simulink model "P2PHVDCMMC"  (R2024a)
settings: Solver=FixedStepDiscrete  StartTime=0.0  StopTime=10  RelTol=1e-3
PreLoadFcn:
  | % HVDCMMCInterconnectionParam
StartFcn:
  | tic
StopFcn:
  | toc
values from neighbouring files (symbols this model uses):
  C_PM = 1.758e-3    (= 0.001758)    [P2PHVDCMMCcode.m]
  Cg = 50e-9    (= 5e-08)    [P2PHVDCMMCcode.m]
  Fc = Fnom*3.37    (= 168.5)    [P2PHVDCMMCcode.m]
  Fnom = 50    [P2PHVDCMMCcode.m]
  HRM = 1    [P2PHVDCMMCcode.m]
  Ki_Ireg = 6    [P2PHVDCMMCcode.m]
  Ki_Preg = 1.0    (= 1)    [P2PHVDCMMCcode.m]
  Ki_Qreg = 1.0    (= 1)    [P2PHVDCMMCcode.m]
  Ki_VDCreg = 100    [P2PHVDCMMCcode.m]
  Kp_Ireg = 0.6    [P2PHVDCMMCcode.m]
  Kp_Preg = 0.5/3    (= 0.166666666667)    [P2PHVDCMMCcode.m]
  Kp_Qreg = 0.5/3    (= 0.166666666667)    [P2PHVDCMMCcode.m]
  Kp_VDCreg = 4    [P2PHVDCMMCcode.m]
  L_cable = 15e-3    (= 0.015)    [P2PHVDCMMCcode.m]
  Larm = Larm_pu*(Zb_ac/(2*pi*Fnom))    [P2PHVDCMMCcode.m]
  Larm_pu = 0.15    [P2PHVDCMMCcode.m]
  Lff = Larm_pu/2    (= 0.075)    [P2PHVDCMMCcode.m]
  Limits_Ireg = [ 2.0  -2.0]    [P2PHVDCMMCcode.m]
  Limits_Preg = [ 1.2, 0.8 ]    [P2PHVDCMMCcode.m]
  Limits_Qreg = [ 0.25, -0.25 ]    [P2PHVDCMMCcode.m]
  Limits_VDCreg = [ 2.0  -2.0]    [P2PHVDCMMCcode.m]
  Lxfo = 0.12    [P2PHVDCMMCcode.m]
  N = 6    [P2PHVDCMMCcode.m]
  Nb_PM = 36    [P2PHVDCMMCcode.m]
  Pnom = 1000e6    (= 1000000000)    [P2PHVDCMMCcode.m]
  R_cable = 0.5    [P2PHVDCMMCcode.m]
  R_startup = 400    [P2PHVDCMMCcode.m]
  Rarm = Rarm_pu*Zb_ac    [P2PHVDCMMCcode.m]
  Rff = Rarm_pu/2    (= 0.00075)    [P2PHVDCMMCcode.m]
  Rg = 100    [P2PHVDCMMCcode.m]
  Rxfo = 0.003    [P2PHVDCMMCcode.m]
  Slope_Qref = 0.5    [P2PHVDCMMCcode.m]
  Slope_Vdc_ref = Vnom_dc/5    (= 128000)    [P2PHVDCMMCcode.m]
  Tfault = 9999    [P2PHVDCMMCcode.m]
  Ts = Ts_Control    (= 4e-05)    [P2PHVDCMMCcode.m]
  Ts_Control = 40e-6    (= 4e-05)    [P2PHVDCMMCcode.m]
  Ts_dqn = 2e-5    (= 2e-05)    [P2PHVDCMMCcode.m]
  Ts_Power = 20e-6    (= 2e-05)    [P2PHVDCMMCcode.m]
  Vnom_dc = 640e3    (= 640000)    [P2PHVDCMMCcode.m]
  Vnom_prim = 400e3    (= 400000)    [P2PHVDCMMCcode.m]
  Vnom_sec = 333e3    (= 333000)    [P2PHVDCMMCcode.m]
  Ws = 2*pi*50    (= 314.159265359)    [P2PHVDCMMCcode.m]
undefined symbols (not defined in the file or in its folder): DiscIntNeverNeededParam, Discrete, DQN_Lib, gcbh, Int_DQNc_Mat, Mult_DQNc_Mat, Pcc, S, sps, sps_rtmsupport, spsMeanValueVariableFrequencyModel, spsPLL3phModel, SY3
libraries: simulink x38, spsControlledVoltageSourceLib x30, spsVoltageMeasurementLib x21, spsIdealSwitchLib x21, powerlib_extras x12, spsSecondOrderFilterLib x12, spsCurrentMeasurementLib x12, spsdq0toabcLib x9, spsMeanLib x8, spsMeanVariableFrequencyLib x8, spsabctodq0Lib x8, spsThreePhaseSeriesRLCBranchLib x7
(part 1 of 13)
settings Model: SimulationMode=accelerator  Creator=The MathWorks, Inc.  LastModifiedBy=salsarayreh
settings SolverCC: AlgebraicLoopSolver=TrustRegion  AutoInsertRateTranBlk=on
settings DataIOCC: SaveFormat=StructureWithTime  SaveOutput=off  DSMLogging=off  SaveTime=off  ReturnWorkspaceOutputs=off
settings OptimizationCC: ReuseModelBlockBuffer=off  ExpressionDepthLimit=2147483647  LifeSpan=inf
settings DebuggingCC: UnderspecifiedInitializationDetection=Classic  MergeDetectMultiDrivingBlocksExec=none  SolverPrmCheckMsg=warning  MultiTaskRateTransMsg=warning  FcnCallInpInsideContextMsg=warning  UnconnectedInputMsg=warning  UnconnectedOutputMsg=warning  UnconnectedLineMsg=warning  AllowSymbolicDim=off  StateNameClashWarn=warning  SFUnexpectedBacktrackingDiag=warning  SFNoUnconditionalDefaultTransitionDiag=warning  SFExecutionAtInitializationDiag=none  ArithmeticOperatorsInVariantConditions=warning
settings HardwareCC: ProdBitPerPointer=32  ProdBitPerSizeT=32  ProdBitPerPtrDiffT=32  ProdLargestAtomicFloat=None  ProdIntDivRoundTo=Undefined  ProdEndianess=Unspecified  ProdWordSize=32  ProdHWDeviceType=32-bit Generic
settings ModelReferenceCC: EnableRefExpFcnMdlSchedulingChecks=on  PropagateSignalLabelsOutOfModel=off
settings SFSimCC: SimUseLocalCustomCode=off  CustomCodeUndefinedFunction=UseInterfaceOnly
settings RTWCC: RTWUseLocalCustomCode=off  GPUComputeCapability=3.5
settings CodeAppCC: StateflowObjectComments=on
settings GRTTargetCC: TargetLangStandard=C89/C90 (ANSI)  CombineOutputUpdateFcns=off  GRTInterface=on
settings ConfigComp: CovMetricSettings=dw  CovSaveCumulativeToWorkspaceVar=on  CovSaveSingleToWorkspaceVar=on  CovExternalEMLEnable=off
settings SimscapeCC: SimscapeNormalizeSystem=off

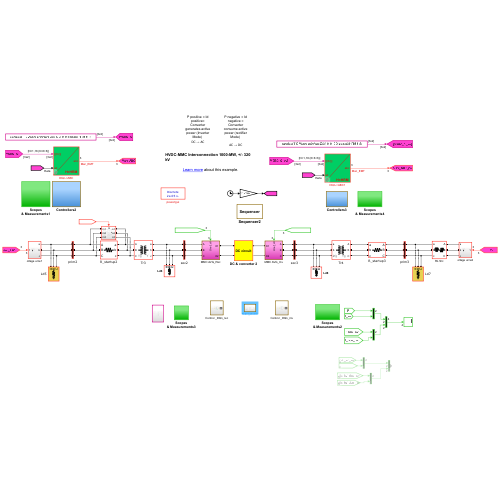
[thumbnail: Simulink's stored preview of the top-level diagram]
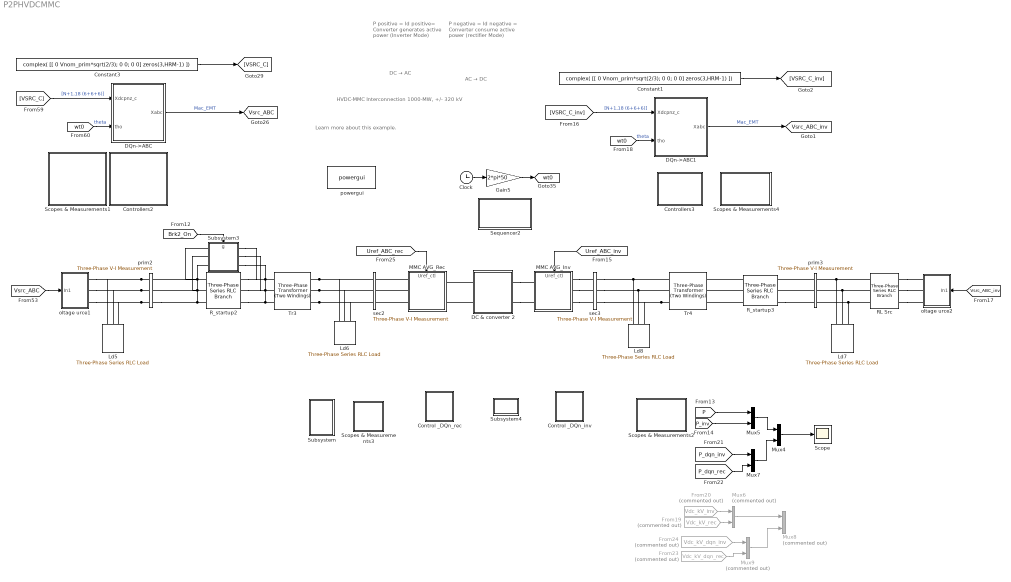
== system P2PHVDCMMC ==
  note: DC → AC
  note: HVDC-MMC Interconnection 1000-MW, +/- 320 kV
  note: Learn more about this example.
  note: P positive = Id positive= Converter generates active power (Inverter Mode)
  note: P negative = Id negative = Converter consume active power (rectifier Mode)
  note: AC → DC
  Clock : Clock
  Constant1 : Constant  Value=complex( [[ 0 Vnom_prim*sqrt(2/3); 0 0; 0 0] zeros(3,HRM-1) ])
  Constant3 : Constant  Value=complex( [[ 0 Vnom_prim*sqrt(2/3); 0 0; 0 0] zeros(3,HRM-1) ])
  Control _DQn_inv : Subsystem
  Control _DQn_rec : Subsystem
  Controllers2 : Subsystem
  Controllers3 : Subsystem
  DC & converter 2 : Subsystem
      mask Display: disp('DC circuit')
  DQn->ABC : MATLAB Function  TreatAsAtomicUnit=on  SystemSampleTime=Ts_Power  mask{N=HRM}
      mask prompts: N "Harmonic order:"
  DQn->ABC1 : MATLAB Function  TreatAsAtomicUnit=on  SystemSampleTime=Ts_Power  mask{N=HRM}
      mask prompts: N "Harmonic order:"
  From19 : From  Commented=on  GotoTag=Vdc_kV_rec  TagVisibility=global
  From20 : From  Commented=on  GotoTag=Vdc_kV_inv  TagVisibility=global
  From23 : From  Commented=on  GotoTag=Vdc_kV_dqn_rec  TagVisibility=global
  From24 : From  Commented=on  GotoTag=Vdc_kV_dqn_inv  TagVisibility=global
  Gain5 : Gain  Gain=2*pi*50
  Ld5 : spsThreePhaseSeriesRLCLoadLib/Three-Phase Series RLC Load  LConnTagsString=A|B|C  Configuration=Y (grounded)  NominalVoltage=Vnom_prim  Vabc=[1e3 1e3 1e3]  Vabcp=[1e3 1e3 1e3]  NominalFrequency=Fnom  UnbalancedPower=off  ActivePower=P_Ld1  InductivePower=0  CapacitivePower=0  Pabc=[10e3 9e3 11e3]  QLabc=[100 90 110]  QCabc=[100 90 110]  Pabcp=[10e3 9e3 11e3]  QLabcp=[100 90 110]  QCabcp=[100 90 110]  Measurements=None  LoadType=constant Z
  Ld6 : spsThreePhaseSeriesRLCLoadLib/Three-Phase Series RLC Load  LConnTagsString=A|B|C  Configuration=Y (grounded)  NominalVoltage=Vnom_sec  Vabc=[1e3 1e3 1e3]  Vabcp=[1e3 1e3 1e3]  NominalFrequency=Fnom  UnbalancedPower=off  ActivePower=500e3  InductivePower=0  CapacitivePower=0  Pabc=[10e3 9e3 11e3]  QLabc=[100 90 110]  QCabc=[100 90 110]  Pabcp=[10e3 9e3 11e3]  QLabcp=[100 90 110]  QCabcp=[100 90 110]  Measurements=None  LoadType=constant Z
  Ld7 : spsThreePhaseSeriesRLCLoadLib/Three-Phase Series RLC Load  LConnTagsString=A|B|C  Configuration=Y (grounded)  NominalVoltage=Vnom_prim  Vabc=[1e3 1e3 1e3]  Vabcp=[1e3 1e3 1e3]  NominalFrequency=Fnom  UnbalancedPower=off  ActivePower=P_Ld1  InductivePower=0  CapacitivePower=0  Pabc=[10e3 9e3 11e3]  QLabc=[100 90 110]  QCabc=[100 90 110]  Pabcp=[10e3 9e3 11e3]  QLabcp=[100 90 110]  QCabcp=[100 90 110]  Measurements=None  LoadType=constant Z
  Ld8 : spsThreePhaseSeriesRLCLoadLib/Three-Phase Series RLC Load  LConnTagsString=A|B|C  Configuration=Y (grounded)  NominalVoltage=Vnom_sec  Vabc=[1e3 1e3 1e3]  Vabcp=[1e3 1e3 1e3]  NominalFrequency=Fnom  UnbalancedPower=off  ActivePower=500e3  InductivePower=0  CapacitivePower=0  Pabc=[10e3 9e3 11e3]  QLabc=[100 90 110]  QCabc=[100 90 110]  Pabcp=[10e3 9e3 11e3]  QLabcp=[100 90 110]  QCabcp=[100 90 110]  Measurements=None  LoadType=constant Z
  MMC AVG_Inv : Subsystem
      settings: PortSchema="{\"entries\":[{\"content\":{\"sides\":[{\"content\":{\"connectorIds\":[\"LConn1\",\"LConn2\",\"LConn3\"]},\"type\":\"ConnectorPlacement.EquallySpacedRectSide\",\"uuid\":\"ba64873c-b22b-410d-af4d-7ba2fdc55c23\"},{\"content\":{\"connectorIds\":[\"RConn1\",\"RConn2\"],\"side\":\"RIGHT\"},\"type\":\"ConnectorPlacement.EquallySpacedRectSide\",\"uuid\":\"193af711-64d0-4e3f-b9d8-3af97f0f6abc\"},{\"content\":{\"connectorIds\":[\"In1\"],\"side\":\"TOP\"},\"type\":\"ConnectorPlacement.EquallySpacedRectSide\",\"uuid\":\"04826a8d-a462-403d-873f-6ac7e8481113\"}]},\"type\":\"ConnectorPlacement.EquallySpacedConnector\",\"uuid\":\"1def47fd-2da9-40af-b501-c2103dcb1fab\"}],\"packageUris\":[\"http://schema.mathworks.com/mf0/Connector/R2020b\"],\"version\":\"1.0\"}"
  MMC AVG_Rec : Subsystem
      settings: PortSchema="{\"entries\":[{\"content\":{\"sides\":[{\"content\":{\"connectorIds\":[\"LConn1\",\"LConn2\",\"LConn3\"]},\"type\":\"ConnectorPlacement.EquallySpacedRectSide\",\"uuid\":\"ba64873c-b22b-410d-af4d-7ba2fdc55c23\"},{\"content\":{\"connectorIds\":[\"RConn1\",\"RConn2\"],\"side\":\"RIGHT\"},\"type\":\"ConnectorPlacement.EquallySpacedRectSide\",\"uuid\":\"193af711-64d0-4e3f-b9d8-3af97f0f6abc\"},{\"content\":{\"connectorIds\":[\"In1\"],\"side\":\"TOP\"},\"type\":\"ConnectorPlacement.EquallySpacedRectSide\",\"uuid\":\"04826a8d-a462-403d-873f-6ac7e8481113\"}]},\"type\":\"ConnectorPlacement.EquallySpacedConnector\",\"uuid\":\"1def47fd-2da9-40af-b501-c2103dcb1fab\"}],\"packageUris\":[\"http://schema.mathworks.com/mf0/Connector/R2020b\"],\"version\":\"1.0\"}"
  Mux4 : Mux  Inputs=2
  Mux5 : Mux  Inputs=2
  Mux6 : Mux  Commented=on  Inputs=2
  Mux7 : Mux  Inputs=2
  Mux8 : Mux  Commented=on  Inputs=2
  Mux9 : Mux  Commented=on  Inputs=2
  RL Src : spsThreePhaseSeriesRLCBranchLib/Three-Phase Series RLC Branch  LConnTagsString=A|B|C  RConnTagsString=A|B|C  BranchType=RL  Resistance=0.8929  Inductance=16.58e-3  Capacitance=1e-6  Measurements=None
  R_startup2 : spsThreePhaseSeriesRLCBranchLib/Three-Phase Series RLC Branch  LConnTagsString=A|B|C  RConnTagsString=A|B|C  BranchType=R  Resistance=R_startup  Inductance=Vnom_prim^2 / Pcc / (2*pi*Fnom)  Capacitance=1e-6  Measurements=None
  R_startup3 : spsThreePhaseSeriesRLCBranchLib/Three-Phase Series RLC Branch  LConnTagsString=A|B|C  RConnTagsString=A|B|C  BranchType=R  Resistance=R_startup/5  Inductance=Vnom_prim^2 / Pcc / (2*pi*Fnom)  Capacitance=1e-6  Measurements=None
  Scope : Scope
  Scopes & Measurements1 : Subsystem
  Scopes & Measurements2 : Subsystem
  Scopes & Measurements3 : Subsystem
  Scopes & Measurements4 : Subsystem
  Sequencer2 : Subsystem
      mask Display: disp('Sequencer')
  Subsystem : Subsystem
  Subsystem3 : Subsystem
      settings: PortSchema="{\"entries\":[{\"content\":{\"sides\":[{\"content\":{\"connectorIds\":[\"LConn1\",\"LConn2\",\"LConn3\"]},\"type\":\"ConnectorPlacement.EquallySpacedRectSide\",\"uuid\":\"c1a766f8-ff9e-46aa-a021-7821e1e68416\"},{\"content\":{\"connectorIds\":[\"RConn1\",\"RConn2\",\"RConn3\"],\"side\":\"RIGHT\"},\"type\":\"ConnectorPlacement.EquallySpacedRectSide\",\"uuid\":\"987c4934-70c2-4017-a470-918577d5d1f5\"},{\"content\":{\"connectorIds\":[\"In1\"],\"side\":\"TOP\"},\"type\":\"ConnectorPlacement.EquallySpacedRectSide\",\"uuid\":\"288129dd-9593-42f2-8eec-9a4ff51cc6bc\"}]},\"type\":\"ConnectorPlacement.EquallySpacedConnector\",\"uuid\":\"6c6a961f-0497-41f0-a1bb-4cb9411a874b\"}],\"packageUris\":[\"http://schema.mathworks.com/mf0/Connector/R2020b\"],\"version\":\"1.0\"}"
  Subsystem4 : Subsystem
  Tr3 : spsThreePhaseTransformerTwoWindingsLib/Three-Phase Transformer (Two Windings)  Winding1Connection=Yg  Winding2Connection=Y  CoreType=Three single-phase transformers  SetSaturation=off  Hysteresis=off  DataFile='hysteresis'  SetInitialFlux=off  Measurements=None  UNITS=pu  NominalPower=[ Pnom , Fnom ]  Winding1="[ Vnom_prim , Rxfo/2,  Lxfo/2 ]"  Winding2="[ Vnom_sec , Rxfo/2,  Lxfo/2 ]"  Rm=1000  Lm=1000  L0=0.5  Saturation=[ 0,0 ; 0.0024,1.2 ; 1.0,1.52 ]  InitialFluxes=[ 0.8 , -0.8 , 0.7 ]  BreakLoop=off  DiscreteSolver=Trapezoidal iterative  DataType=off  TransfoNumber=1
  Tr4 : spsThreePhaseTransformerTwoWindingsLib/Three-Phase Transformer (Two Windings)  Winding1Connection=Yg  Winding2Connection=Yg  CoreType=Three single-phase transformers  SetSaturation=off  Hysteresis=off  DataFile='hysteresis'  SetInitialFlux=off  Measurements=None  UNITS=pu  NominalPower=[ Pnom , Fnom ]  Winding1="[ Vnom_prim , Rxfo/2,  Lxfo/2 ]"  Winding2="[ Vnom_sec , Rxfo/2,  Lxfo/2 ]"  Rm=1000  Lm=1000  L0=0.5  Saturation=[ 0,0 ; 0.0024,1.2 ; 1.0,1.52 ]  InitialFluxes=[ 0.8 , -0.8 , 0.7 ]  BreakLoop=off  DiscreteSolver=Trapezoidal iterative  DataType=off  TransfoNumber=1
  oltage urce1 : Subsystem
  oltage urce2 : Subsystem
  powergui : spspowerguiLib/powergui  Priority=1  SimulationMode=Discrete  SampleTime=Ts_Power  frequency=60  Iterations=50  frequencyindice=0  Pbase=100e6  ErrMax=1e-4  UnitsV=kV  UnitsW=MW  buscounter=0  FunctionMessages=off  echomessages=off  EnableUseOfTLC=off  CurrentSourceSwitches=off  DisableSnubberDevices=off  DisableRonSwitches=off  DisableVfSwitches=off  DisplayEquations=off  AutomaticDiscreteSolvers=off  SolverType=Tustin/Backward Euler (TBE)  Interpol=off  ExternalGateDelay=off  methode=off  Ts=10  x0status=blocks  SPID=off  SwTol=0  HookPort=off  NonlinearTolerance=1e-4  nMaxIteration=100  ContinueOnMaxIteration=off  RestoreLinks=warning  ResistiveCurrentMeasurement=off  Frange=[0:2:500]  Ylog=off  Xlog=on  ShowGrid=off  save=off  variable=ZData  structure=VIprim  ZoomFFT=on  StartTime=0.15  cycles=2  DisplayStyle=1  fundamental=50  FreqAxis=on  MaxFrequency=1000  frequencyindicesteady=1  RmsSteady=1  display=off
  prim2 : spsThreePhaseVIMeasurementLib/Three-Phase V-I Measurement  VoltageMeasurement=phase-to-ground  SetLabelV=on  LabelV=Vprim  Vpu=off  VpuLL=off  CurrentMeasurement=yes  SetLabelI=on  LabelI=Iprim  Ipu=off  Pbase=100e6  Vbase=500e3  OutputType=Complex  PhasorSimulation=off  PSBequivalent=0
  prim3 : spsThreePhaseVIMeasurementLib/Three-Phase V-I Measurement  VoltageMeasurement=phase-to-ground  SetLabelV=on  LabelV=Vprim_inv  Vpu=off  VpuLL=off  CurrentMeasurement=yes  SetLabelI=on  LabelI=Iprim_inv  Ipu=off  Pbase=100e6  Vbase=500e3  OutputType=Complex  PhasorSimulation=off  PSBequivalent=0
  sec2 : spsThreePhaseVIMeasurementLib/Three-Phase V-I Measurement  VoltageMeasurement=phase-to-ground  SetLabelV=on  LabelV=Vsec  Vpu=off  VpuLL=off  CurrentMeasurement=yes  SetLabelI=on  LabelI=Isec  Ipu=off  Pbase=100e6  Vbase=500e3  OutputType=Complex  PhasorSimulation=off  PSBequivalent=0
  sec3 : spsThreePhaseVIMeasurementLib/Three-Phase V-I Measurement  VoltageMeasurement=phase-to-ground  SetLabelV=on  LabelV=Vsec_inv  Vpu=off  VpuLL=off  CurrentMeasurement=yes  SetLabelI=on  LabelI=Isec_inv  Ipu=off  Pbase=100e6  Vbase=500e3  OutputType=Complex  PhasorSimulation=off  PSBequivalent=0
  tag scope: Vsrc_ABC=global, Vsrc_ABC_inv=global, wt0=global
  wires:
  [Vsrc_ABC] -> oltage urce1/1(In1)
  Gain5/1 -> [wt0]
  [Uref_ABC_rec] -> MMC AVG_Rec/1(Uref_ctl)
  [VSRC_C] -> DQn->ABC/1(Xdcpnz_c)  "[N+1,18 (6+6+6)]"
  [wt0] -> DQn->ABC/2(tho)  "theta"
  Constant3/1 -> [VSRC_C]
  Clock/1 -> Gain5/1
  DQn->ABC/1(Xabc) -> [Vsrc_ABC]  "Mac_EMT"
  [Brk2_On] -> Subsystem3/1(g)
  [Vsrc_ABC_inv] -> oltage urce2/1(In1)
  [Uref_ABC_inv] -> MMC AVG_Inv/1(Uref_ctl)
  [wt0] -> DQn->ABC1/2(tho)  "theta"
  Constant1/1 -> [VSRC_C_inv]
  [VSRC_C_inv] -> DQn->ABC1/1(Xdcpnz_c)  "[N+1,18 (6+6+6)]"
  DQn->ABC1/1(Xabc) -> [Vsrc_ABC_inv]  "Mac_EMT"
  [P] -> Mux5/1
  [P_inv] -> Mux5/2
  Mux5/1 -> Mux4/1
  Mux4/1 -> Scope/1
  Mux6/1 -> Mux8/1
  From19/1 -> Mux6/2
  From20/1 -> Mux6/1
  [P_dqn_rec] -> Mux7/2
  [P_dqn_inv] -> Mux7/1
  Mux7/1 -> Mux4/2
  From24/1 -> Mux9/1
  From23/1 -> Mux9/2
  Mux9/1 -> Mux8/2
  connections:
  Tr3/RConn2 -- sec2/RConn2 -- Ld6/LConn2
  Tr3/RConn1 -- sec2/RConn1 -- Ld6/LConn1
  Tr3/RConn3 -- sec2/RConn3 -- Ld6/LConn3
  Tr3/LConn2 -- Subsystem3/RConn2 -- R_startup2/RConn2
  R_startup2/LConn2 -- Subsystem3/LConn2 -- prim2/LConn2
  R_startup2/LConn3 -- Subsystem3/LConn3 -- prim2/LConn3
  Tr3/LConn1 -- Subsystem3/RConn1 -- R_startup2/RConn1
  Tr3/LConn3 -- Subsystem3/RConn3 -- R_startup2/RConn3
  R_startup2/LConn1 -- Subsystem3/LConn1 -- prim2/LConn1
  prim2/RConn1 -- Ld5/LConn1 -- oltage urce1/RConn1
  prim2/RConn3 -- Ld5/LConn3 -- oltage urce1/RConn3
  prim2/RConn2 -- Ld5/LConn2 -- oltage urce1/RConn2
  MMC AVG_Rec/LConn1 -- sec2/LConn1
  DC & converter 2/LConn2 -- MMC AVG_Rec/RConn2
  MMC AVG_Rec/LConn2 -- sec2/LConn2
  MMC AVG_Rec/LConn3 -- sec2/LConn3
  DC & converter 2/LConn1 -- MMC AVG_Rec/RConn1
  Tr4/RConn3 -- sec3/RConn3 -- Ld8/LConn3
  RL Src/RConn1 -- Ld7/LConn1 -- prim3/RConn1
  prim3/LConn2 -- R_startup3/LConn2
  RL Src/RConn3 -- Ld7/LConn3 -- prim3/RConn3
  R_startup3/RConn1 -- Tr4/LConn1
  R_startup3/RConn3 -- Tr4/LConn3
  RL Src/RConn2 -- Ld7/LConn2 -- prim3/RConn2
  sec3/RConn1 -- Ld8/LConn1 -- Tr4/RConn1
  R_startup3/LConn3 -- prim3/LConn3
  prim3/LConn1 -- R_startup3/LConn1
  R_startup3/RConn2 -- Tr4/LConn2
  sec3/RConn2 -- Ld8/LConn2 -- Tr4/RConn2
  RL Src/LConn3 -- oltage urce2/RConn3
  MMC AVG_Inv/LConn2 -- sec3/LConn2
  MMC AVG_Inv/LConn3 -- sec3/LConn3
  MMC AVG_Inv/LConn1 -- sec3/LConn1
  RL Src/LConn1 -- oltage urce2/RConn1
  RL Src/LConn2 -- oltage urce2/RConn2
  DC & converter 2/RConn1 -- MMC AVG_Inv/RConn1
  DC & converter 2/RConn2 -- MMC AVG_Inv/RConn2

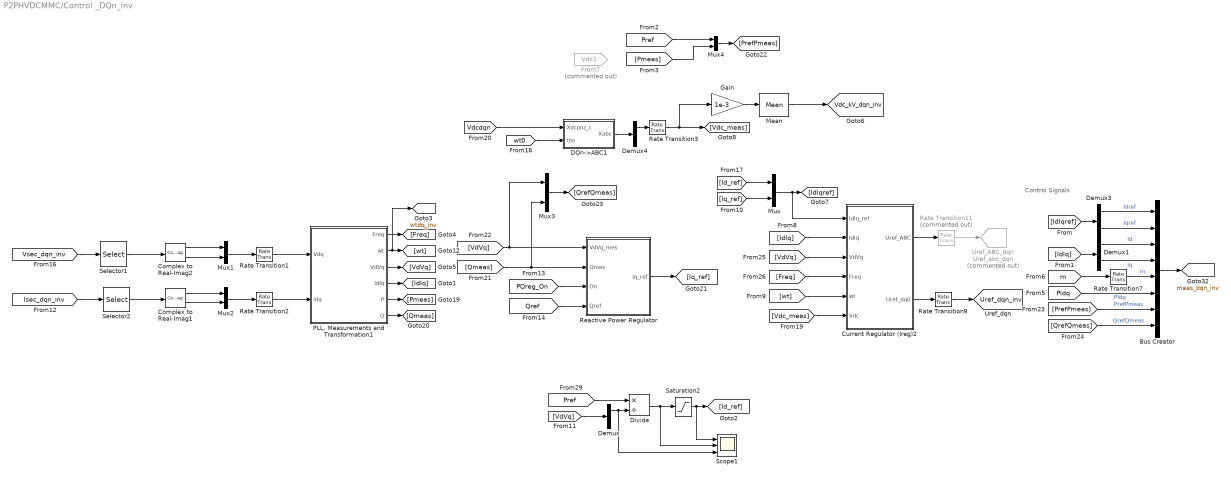
== system P2PHVDCMMC/Control _DQn_inv ==
  note: Control Signals
  Bus Creator : BusCreator  Inputs=8
  Complex to Real-Imag1 : ComplexToRealImag
  Complex to Real-Imag2 : ComplexToRealImag
  Current Regulator (Ireg)2 : Subsystem
  DQn->ABC1 : MATLAB Function  TreatAsAtomicUnit=on  SystemSampleTime=Ts_Power  mask{N=N+3}
      mask prompts: N "Harmonic order:"
  Demux : Demux  Outputs=2
  Demux1 : Demux  Outputs=2
  Demux3 : Demux  Outputs=2
  Demux4 : Demux  Outputs=3
  Divide : Product  Inputs=*/
  From7 : From  Commented=on  GotoTag=Vdc1  TagVisibility=global
  Gain : Gain  Gain=1e-3
  Mean : spsMeanLib/Mean  Freq=Fnom/3  Vinit=0  Ts=Ts_Control
  Mux{,1..4} (5 alike) : Mux  Inputs=2
  "PLL, Measurements and Transformation1" : Subsystem
  Rate Transition{1..3,7} (4 alike) : RateTransition  OutPortSampleTime=Ts_Control
  Rate Transition11 : RateTransition  Commented=on  OutPortSampleTime=Ts_Power
  Rate Transition9 : RateTransition  OutPortSampleTime=Ts_Power
  Reactive Power Regulator : Subsystem
  Saturation2 : Saturate  UpperLimit=Limits_VDCreg(1)  LowerLimit=Limits_VDCreg(2)  SampleTime=Ts
  Scope1 : Scope  NumInputPorts=3
  Selector1 : Selector  NumberOfDimensions=2  InputPortWidth=3  IndexOptions=Index vector (dialog),Index vector (dialog)  Indices=1,2  OutputSizes=1,1
  Selector2 : Selector  NumberOfDimensions=2  InputPortWidth=3  IndexOptions=Index vector (dialog),Index vector (dialog)  Indices=1,2  OutputSizes=1,1
  Uref_ABC_dqn : Goto  Commented=on  GotoTag=Uref_abc_dqn  TagVisibility=global
  tag scope: Uref_dqn_inv=global, Vdc_kV_dqn_inv=global, meas_dqn_inv=global, wtdq_inv=global
  wires:
  Complex to Real-Imag2/1 -> Mux1/1
  [PQreg_On] -> Reactive Power Regulator/3(On)
  Selector1/1 -> Complex to Real-Imag2/1
  Complex to Real-Imag2/2 -> Mux1/2
  [Vsec_dqn_inv] -> Selector1/1
  [Qref] -> Reactive Power Regulator/4(Qref)
  Complex to Real-Imag1/2 -> Mux2/2
  Selector2/1 -> Complex to Real-Imag1/1
  Complex to Real-Imag1/1 -> Mux2/1
  [Isec_dqn_inv] -> Selector2/1
  Current Regulator (Ireg)2/1(Uref_ABC) -> Rate Transition11/1
  Mux1/1 -> Rate Transition1/1
  Mux2/1 -> Rate Transition2/1
  Rate Transition1/1 -> "PLL, Measurements and Transformation1"/1(Vdq)
  Rate Transition2/1 -> "PLL, Measurements and Transformation1"/2(Idq)
  Rate Transition11/1 -> Uref_ABC_dqn/1
  [PrefPmeas] -> Bus Creator/7  "PrefPmeas"
  [Pref] -> Mux4/1
  [QrefQmeas] -> Bus Creator/8  "QrefQmeas"
  Mux4/1 -> [PrefPmeas]
  Gain/1 -> Mean/1
  [Pmeas] -> Mux4/2
  [m] -> Rate Transition7/1
  Rate Transition3/1 -> Gain/1, [Vdc_meas]
  Demux3/1 -> Bus Creator/1  "Idref"
  Rate Transition7/1 -> Bus Creator/5  "m"
  [IdIq] -> Demux1/1
  Bus Creator/1 -> [meas_dqn_inv]
  Demux1/1 -> Bus Creator/3  "Id"
  Demux3/2 -> Bus Creator/2  "Iqref"
  [IdIqref] -> Demux3/1
  [PIdq] -> Bus Creator/6  "PIdq"
  [Id_ref] -> Mux/1
  Demux1/2 -> Bus Creator/4  "Iq"
  [Iq_ref] -> Mux/2
  Mean/1 -> [Vdc_kV_dqn_inv]
  "PLL, Measurements and Transformation1"/6(Q) -> [Qmeas]
  "PLL, Measurements and Transformation1"/5(P) -> [Pmeas]
  "PLL, Measurements and Transformation1"/4(IdIq) -> [IdIq]
  "PLL, Measurements and Transformation1"/3(VdVq) -> [VdVq]
  "PLL, Measurements and Transformation1"/2(wt) -> [wtdq_inv], [wt]
  "PLL, Measurements and Transformation1"/1(Freq) -> [Freq]
  Reactive Power Regulator/1(Iq_ref) -> [Iq_ref]
  [Qmeas] -> Mux3/2, Reactive Power Regulator/2(Qmes)
  [VdVq] -> Mux3/1, Reactive Power Regulator/1(VdVq_mes)
  Mux3/1 -> [QrefQmeas]
  Mux/1 -> Current Regulator (Ireg)2/1(IdIq_ref), [IdIqref]
  [IdIq] -> Current Regulator (Ireg)2/2(IdIq)
  [VdVq] -> Current Regulator (Ireg)2/3(VdVq)
  [wt] -> Current Regulator (Ireg)2/5(wt)
  [Freq] -> Current Regulator (Ireg)2/4(Freq)
  [Vdc_meas] -> Current Regulator (Ireg)2/6(Vdc)
  Current Regulator (Ireg)2/2(Uref_dq0) -> Rate Transition9/1
  Rate Transition9/1 -> [Uref_dqn_inv]
  Demux/1 -> Scope1/3, Divide/2
  Saturation2/1 -> Scope1/1, [Id_ref]
  Divide/1 -> Scope1/2, Saturation2/1
  [Pref] -> Divide/1
  [VdVq] -> Demux/1
  [wt0] -> DQn->ABC1/2(tho)
  Demux4/1 -> Rate Transition3/1
  [Vdcdqn] -> DQn->ABC1/1(Xdcpnz_c)
  DQn->ABC1/1(Xabc) -> Demux4/1

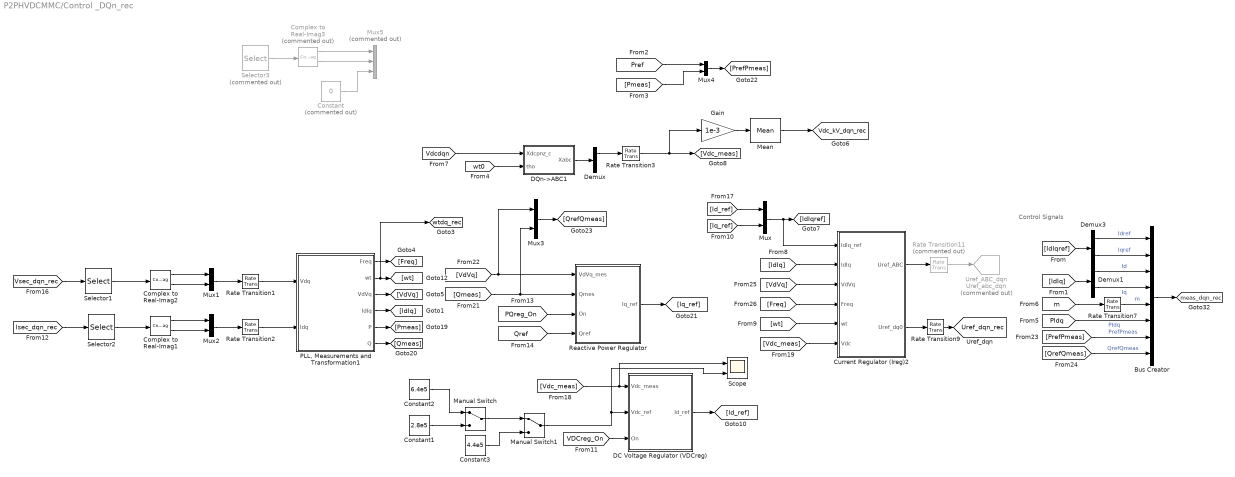
== system P2PHVDCMMC/Control _DQn_rec ==
  note: Control Signals
  Bus Creator : BusCreator  Inputs=8
  Complex to Real-Imag1 : ComplexToRealImag
  Complex to Real-Imag2 : ComplexToRealImag
  Complex to Real-Imag3 : ComplexToRealImag  Commented=on
  Constant : Constant  Commented=on  Value=0
  Constant1 : Constant  Value=2.8e5  SampleTime=Ts_Control
  Constant2 : Constant  Value=6.4e5  SampleTime=Ts_Control
  Constant3 : Constant  Value=4.4e5  SampleTime=Ts_Control
  Current Regulator (Ireg)2 : Subsystem
  DC Voltage Regulator (VDCreg) : Subsystem
  DQn->ABC1 : MATLAB Function  TreatAsAtomicUnit=on  SystemSampleTime=Ts_Power  mask{N=N+3}
      mask prompts: N "Harmonic order:"
  Demux : Demux  Outputs=3
  Demux1 : Demux  Outputs=2
  Demux3 : Demux  Outputs=2
  Gain : Gain  Gain=1e-3
  Manual Switch : ManualSwitch
  Manual Switch1 : ManualSwitch
  Mean : spsMeanLib/Mean  Freq=Fnom/3  Vinit=0  Ts=Ts_Control
  Mux{,1..4} (5 alike) : Mux  Inputs=2
  Mux5 : Mux  Commented=on  Inputs=3
  "PLL, Measurements and Transformation1" : Subsystem
  Rate Transition{1..3,7} (4 alike) : RateTransition  OutPortSampleTime=Ts_Control
  Rate Transition11 : RateTransition  Commented=on  OutPortSampleTime=Ts_Power
  Rate Transition9 : RateTransition  OutPortSampleTime=Ts_Power
  Reactive Power Regulator : Subsystem
  Scope : Scope  NumInputPorts=2
  Selector1 : Selector  NumberOfDimensions=2  InputPortWidth=3  IndexOptions=Index vector (dialog),Index vector (dialog)  Indices=1,2  OutputSizes=1,1
  Selector2 : Selector  NumberOfDimensions=2  InputPortWidth=3  IndexOptions=Index vector (dialog),Index vector (dialog)  Indices=1,2  OutputSizes=1,1
  Selector3 : Selector  Commented=on  NumberOfDimensions=2  InputPortWidth=3  IndexOptions=Index vector (dialog),Index vector (dialog)  Indices=3,1  OutputSizes=1,1
  Uref_ABC_dqn : Goto  Commented=on  GotoTag=Uref_abc_dqn  TagVisibility=global
  tag scope: Uref_dqn_rec=global, Vdc_kV_dqn_rec=global, meas_dqn_rec=global, wtdq_rec=global
  wires:
  Complex to Real-Imag2/1 -> Mux1/1
  [PQreg_On] -> Reactive Power Regulator/3(On)
  Selector1/1 -> Complex to Real-Imag2/1
  Complex to Real-Imag2/2 -> Mux1/2
  [Vsec_dqn_rec] -> Selector1/1
  [Qref] -> Reactive Power Regulator/4(Qref)
  Complex to Real-Imag1/2 -> Mux2/2
  Selector2/1 -> Complex to Real-Imag1/1
  Complex to Real-Imag1/1 -> Mux2/1
  [Isec_dqn_rec] -> Selector2/1
  Current Regulator (Ireg)2/1(Uref_ABC) -> Rate Transition11/1
  Mux1/1 -> Rate Transition1/1
  Mux2/1 -> Rate Transition2/1
  Rate Transition1/1 -> "PLL, Measurements and Transformation1"/1(Vdq)
  Rate Transition2/1 -> "PLL, Measurements and Transformation1"/2(Idq)
  Rate Transition11/1 -> Uref_ABC_dqn/1
  [PrefPmeas] -> Bus Creator/7  "PrefPmeas"
  [Pref] -> Mux4/1
  [QrefQmeas] -> Bus Creator/8  "QrefQmeas"
  Mux4/1 -> [PrefPmeas]
  Gain/1 -> Mean/1
  [Pmeas] -> Mux4/2
  [m] -> Rate Transition7/1
  Rate Transition3/1 -> Gain/1, [Vdc_meas]
  Demux3/1 -> Bus Creator/1  "Idref"
  Rate Transition7/1 -> Bus Creator/5  "m"
  [IdIq] -> Demux1/1
  Bus Creator/1 -> [meas_dqn_rec]
  Demux1/1 -> Bus Creator/3  "Id"
  Demux3/2 -> Bus Creator/2  "Iqref"
  [IdIqref] -> Demux3/1
  [PIdq] -> Bus Creator/6  "PIdq"
  [Id_ref] -> Mux/1
  Demux1/2 -> Bus Creator/4  "Iq"
  DQn->ABC1/1(Xabc) -> Demux/1
  [Iq_ref] -> Mux/2
  Mean/1 -> [Vdc_kV_dqn_rec]
  "PLL, Measurements and Transformation1"/6(Q) -> [Qmeas]
  "PLL, Measurements and Transformation1"/5(P) -> [Pmeas]
  "PLL, Measurements and Transformation1"/4(IdIq) -> [IdIq]
  "PLL, Measurements and Transformation1"/3(VdVq) -> [VdVq]
  "PLL, Measurements and Transformation1"/2(wt) -> [wtdq_rec], [wt]
  "PLL, Measurements and Transformation1"/1(Freq) -> [Freq]
  Reactive Power Regulator/1(Iq_ref) -> [Iq_ref]
  [Qmeas] -> Mux3/2, Reactive Power Regulator/2(Qmes)
  [VdVq] -> Mux3/1, Reactive Power Regulator/1(VdVq_mes)
  Mux3/1 -> [QrefQmeas]
  Mux/1 -> Current Regulator (Ireg)2/1(IdIq_ref), [IdIqref]
  [IdIq] -> Current Regulator (Ireg)2/2(IdIq)
  [VdVq] -> Current Regulator (Ireg)2/3(VdVq)
  [wt] -> Current Regulator (Ireg)2/5(wt)
  [Freq] -> Current Regulator (Ireg)2/4(Freq)
  [Vdc_meas] -> Current Regulator (Ireg)2/6(Vdc)
  Current Regulator (Ireg)2/2(Uref_dq0) -> Rate Transition9/1
  Rate Transition9/1 -> [Uref_dqn_rec]
  Constant3/1 -> Manual Switch1/2
  Constant1/1 -> Manual Switch/2
  Constant2/1 -> Manual Switch/1
  DC Voltage Regulator (VDCreg)/1(Id_ref) -> [Id_ref]
  Manual Switch/1 -> Manual Switch1/1
  [Vdc_meas] -> Scope/1, DC Voltage Regulator (VDCreg)/1(Vdc_meas)
  Manual Switch1/1 -> Scope/2, DC Voltage Regulator (VDCreg)/2(Vdc_ref)
  [VDCreg_On] -> DC Voltage Regulator (VDCreg)/3(On)
  Complex to Real-Imag3/1 -> Mux5/1
  Complex to Real-Imag3/2 -> Mux5/2
  Selector3/1 -> Complex to Real-Imag3/1
  [Vdcdqn] -> DQn->ABC1/1(Xdcpnz_c)
  Constant/1 -> Mux5/3
  Demux/1 -> Rate Transition3/1
  [wt0] -> DQn->ABC1/2(tho)

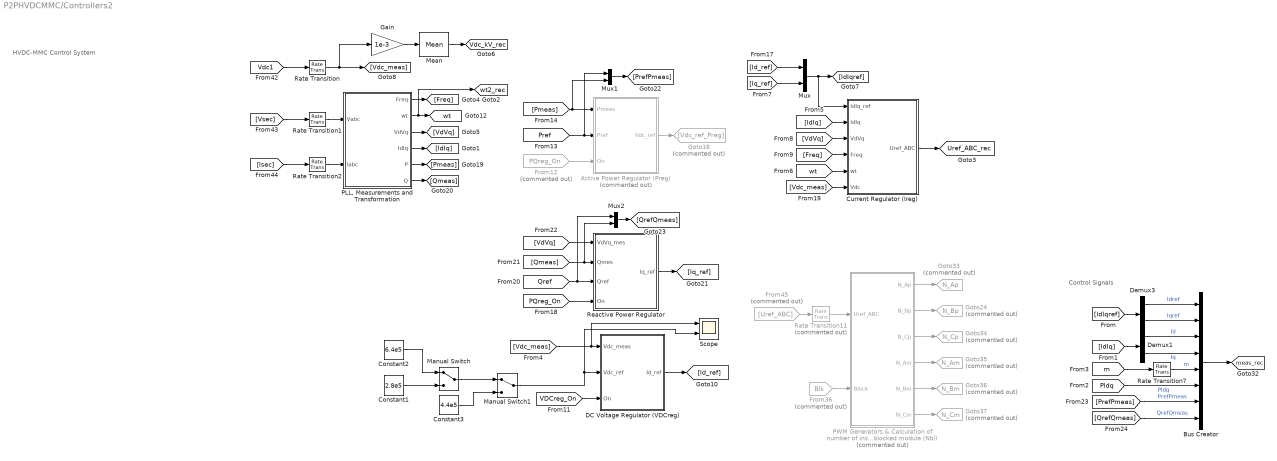
== system P2PHVDCMMC/Controllers2 ==
  note: HVDC-MMC Control System
  note: Control Signals
  Active Power Regulator (Preg) : Subsystem  Commented=on
  Bus Creator : BusCreator  Inputs=8
  Constant1 : Constant  Value=2.8e5  SampleTime=Ts_Control
  Constant2 : Constant  Value=6.4e5  SampleTime=Ts_Control
  Constant3 : Constant  Value=4.4e5  SampleTime=Ts_Control
  Current Regulator (Ireg) : Subsystem
  DC Voltage Regulator (VDCreg) : Subsystem
  Demux1 : Demux  Outputs=2
  Demux3 : Demux  Outputs=2
  From12 : From  Commented=on  GotoTag=PQreg_On  TagVisibility=global
  From36 : From  Commented=on  GotoTag=Blk  TagVisibility=global
  From45 : From  Commented=on  GotoTag=Uref_ABC  TagVisibility=global
  Gain : Gain  Gain=1e-3
  Goto18 : Goto  Commented=on  GotoTag=Vdc_ref_Preg
  Goto24 : Goto  Commented=on  GotoTag=N_Bp  TagVisibility=global
  Goto33 : Goto  Commented=on  GotoTag=N_Ap  TagVisibility=global
  Goto34 : Goto  Commented=on  GotoTag=N_Cp  TagVisibility=global
  Goto35 : Goto  Commented=on  GotoTag=N_Am  TagVisibility=global
  Goto36 : Goto  Commented=on  GotoTag=N_Bm  TagVisibility=global
  Goto37 : Goto  Commented=on  GotoTag=N_Cm  TagVisibility=global
  Manual Switch : ManualSwitch
  Manual Switch1 : ManualSwitch
  Mean : spsMeanLib/Mean  Freq=Fnom/3  Vinit=0  Ts=Ts_Control
  Mux : Mux  Inputs=2
  Mux1 : Mux  Inputs=2
  Mux2 : Mux  Inputs=2
  "PLL, Measurements and Transformation" : Subsystem
  PWM Generators & Calculation of number of inserted modules (Nin) and number of blocked module (Nbl) : Subsystem  Commented=on
  Rate Transition{,1..2,7} (4 alike) : RateTransition  OutPortSampleTime=Ts_Control
  Rate Transition11 : RateTransition  Commented=on  OutPortSampleTime=Ts_Power
  Reactive Power Regulator : Subsystem
  Scope : Scope  NumInputPorts=2
  tag scope: Uref_ABC_rec=global, Vdc_kV_rec=global, meas_rec=global, wt2_rec=global, wt=global
  wires:
  Rate Transition11/1 -> PWM Generators & Calculation of number of inserted modules (Nin) and number of blocked module (Nbl)/1(Uref_ABC)
  From45/1 -> Rate Transition11/1
  Mean/1 -> [Vdc_kV_rec]
  [Vsec] -> Rate Transition1/1
  [Isec] -> Rate Transition2/1
  [Vdc_meas] -> Current Regulator (Ireg)/6(Vdc)
  [Vdc_meas] -> Scope/1, DC Voltage Regulator (VDCreg)/1(Vdc_meas)
  DC Voltage Regulator (VDCreg)/1(Id_ref) -> [Id_ref]
  Gain/1 -> Mean/1
  Current Regulator (Ireg)/1(Uref_ABC) -> [Uref_ABC_rec]
  [wt] -> Current Regulator (Ireg)/5(wt)
  [Vdc1] -> Rate Transition/1
  "PLL, Measurements and Transformation"/2(wt) -> [wt], [wt2_rec]
  "PLL, Measurements and Transformation"/4(IdIq) -> [IdIq]
  [Freq] -> Current Regulator (Ireg)/4(Freq)
  [Id_ref] -> Mux/1
  "PLL, Measurements and Transformation"/3(VdVq) -> [VdVq]
  Mux/1 -> Current Regulator (Ireg)/1(IdIq_ref), [IdIqref]
  Demux1/2 -> Bus Creator/4  "Iq"
  [IdIq] -> Current Regulator (Ireg)/2(IdIq)
  [IdIqref] -> Demux3/1
  Demux3/1 -> Bus Creator/1  "Idref"
  [IdIq] -> Demux1/1
  Bus Creator/1 -> [meas_rec]
  Demux3/2 -> Bus Creator/2  "Iqref"
  [m] -> Rate Transition7/1
  Demux1/1 -> Bus Creator/3  "Id"
  [PIdq] -> Bus Creator/6  "PIdq"
  "PLL, Measurements and Transformation"/1(Freq) -> [Freq]
  [VdVq] -> Current Regulator (Ireg)/3(VdVq)
  [Iq_ref] -> Mux/2
  Rate Transition/1 -> Gain/1, [Vdc_meas]
  Rate Transition2/1 -> "PLL, Measurements and Transformation"/2(Iabc)
  Rate Transition7/1 -> Bus Creator/5  "m"
  Rate Transition1/1 -> "PLL, Measurements and Transformation"/1(Vabc)
  [PQreg_On] -> Reactive Power Regulator/4(On)
  Mux2/1 -> [QrefQmeas]
  Mux1/1 -> [PrefPmeas]
  [Qref] -> Mux2/1, Reactive Power Regulator/3(Qref)
  [QrefQmeas] -> Bus Creator/8  "QrefQmeas"
  [VDCreg_On] -> DC Voltage Regulator (VDCreg)/3(On)
  From12/1 -> Active Power Regulator (Preg)/3(On)
  Active Power Regulator (Preg)/1(Vdc_ref) -> Goto18/1
  Reactive Power Regulator/1(Iq_ref) -> [Iq_ref]
  "PLL, Measurements and Transformation"/5(P) -> [Pmeas]
  [VdVq] -> Reactive Power Regulator/1(VdVq_mes)
  [Qmeas] -> Mux2/2, Reactive Power Regulator/2(Qmes)
  [Pref] -> Active Power Regulator (Preg)/2(Pref), Mux1/1
  [PrefPmeas] -> Bus Creator/7  "PrefPmeas"
  "PLL, Measurements and Transformation"/6(Q) -> [Qmeas]
  [Pmeas] -> Active Power Regulator (Preg)/1(Pmeas), Mux1/2
  PWM Generators & Calculation of number of inserted modules (Nin) and number of blocked module (Nbl)/1(N_Ap) -> Goto33/1
  PWM Generators & Calculation of number of inserted modules (Nin) and number of blocked module (Nbl)/2(N_Bp) -> Goto24/1
  PWM Generators & Calculation of number of inserted modules (Nin) and number of blocked module (Nbl)/3(N_Cp) -> Goto34/1
  PWM Generators & Calculation of number of inserted modules (Nin) and number of blocked module (Nbl)/4(N_Am) -> Goto35/1
  PWM Generators & Calculation of number of inserted modules (Nin) and number of blocked module (Nbl)/5(N_Bm) -> Goto36/1
  PWM Generators & Calculation of number of inserted modules (Nin) and number of blocked module (Nbl)/6(N_Cm) -> Goto37/1
  From36/1 -> PWM Generators & Calculation of number of inserted modules (Nin) and number of blocked module (Nbl)/2(Block)
  Manual Switch1/1 -> Scope/2, DC Voltage Regulator (VDCreg)/2(Vdc_ref)
  Constant2/1 -> Manual Switch/1
  Constant1/1 -> Manual Switch/2
  Manual Switch/1 -> Manual Switch1/1
  Constant3/1 -> Manual Switch1/2

== system P2PHVDCMMC/Controllers3 ==
  note: Control Signals
  Bus Creator : BusCreator  Inputs=8
  Constant : Constant  Commented=on  Value=6.4e5
  Current Regulator (Ireg) : Subsystem
  Demux : Demux  Outputs=2
  Demux1 : Demux  Outputs=2
  Demux3 : Demux  Outputs=2
  Divide : Product  Inputs=*/
  Gain : Gain  Gain=1e-3
  Goto9 : Goto  Commented=on  GotoTag=Uref_ABC_dq2  TagVisibility=global
  Mean : spsMeanLib/Mean  Freq=Fnom/3  Vinit=0  Ts=Ts_Control
  Mux : Mux  Inputs=2
  Mux1 : Mux  Inputs=2
  Mux2 : Mux  Inputs=2
  "PLL, Measurements and Transformation" : Subsystem
  Rate Transition{,1..2,7} (4 alike) : RateTransition  OutPortSampleTime=Ts_Control
  Reactive Power Regulator : Subsystem
  Saturation2 : Saturate  UpperLimit=Limits_VDCreg(1)  LowerLimit=Limits_VDCreg(2)  SampleTime=Ts
  Scope1 : Scope  Commented=on
  tag scope: Uref_ABC_inv=global, Vdc_kV_inv=global, meas_inv=global, wt2_inv=global
  wires:
  Mean/1 -> [Vdc_kV_inv]
  [Vsec_inv] -> Rate Transition1/1
  [Isec_inv] -> Rate Transition2/1
  [Vdc_meas] -> Current Regulator (Ireg)/6(Vdc)
  Gain/1 -> Mean/1
  Current Regulator (Ireg)/1(Uref_ABC) -> [Uref_ABC_inv]
  [wt] -> Current Regulator (Ireg)/5(wt)
  [Vdc1] -> Rate Transition/1
  "PLL, Measurements and Transformation"/2(wt) -> [wt2_inv], [wt]
  "PLL, Measurements and Transformation"/4(IdIq) -> [IdIq]
  [Freq] -> Current Regulator (Ireg)/4(Freq)
  [Id_ref] -> Mux/1
  "PLL, Measurements and Transformation"/3(VdVq) -> [VdVq]
  Mux/1 -> Current Regulator (Ireg)/1(IdIq_ref), [IdIqref]
  Demux1/2 -> Bus Creator/4  "Iq"
  [IdIq] -> Current Regulator (Ireg)/2(IdIq)
  [IdIqref] -> Demux3/1
  Demux3/1 -> Bus Creator/1  "Idref"
  [IdIq] -> Demux1/1
  Bus Creator/1 -> [meas_inv]
  Demux3/2 -> Bus Creator/2  "Iqref"
  [m_inv] -> Rate Transition7/1
  Demux1/1 -> Bus Creator/3  "Id"
  [PIdq_inv] -> Bus Creator/6  "PIdq"
  "PLL, Measurements and Transformation"/1(Freq) -> [Freq]
  [VdVq] -> Current Regulator (Ireg)/3(VdVq)
  [Iq_ref] -> Mux/2
  Rate Transition/1 -> Gain/1, [Vdc_meas]
  Rate Transition2/1 -> "PLL, Measurements and Transformation"/2(Iabc)
  Rate Transition7/1 -> Bus Creator/5  "m"
  Rate Transition1/1 -> "PLL, Measurements and Transformation"/1(Vabc)
  [PQreg_On] -> Reactive Power Regulator/4(On)
  Mux2/1 -> [QrefQmeas]
  Mux1/1 -> [PrefPmeas]
  [Qref] -> Mux2/1, Reactive Power Regulator/3(Qref)
  [QrefQmeas] -> Bus Creator/8  "QrefQmeas"
  Reactive Power Regulator/1(Iq_ref) -> [Iq_ref]
  "PLL, Measurements and Transformation"/5(P) -> [Pmeas]
  [VdVq] -> Reactive Power Regulator/1(VdVq_mes)
  [Qmeas] -> Mux2/2, Reactive Power Regulator/2(Qmes)
  [Pref] -> Mux1/1
  [PrefPmeas] -> Bus Creator/7  "PrefPmeas"
  "PLL, Measurements and Transformation"/6(Q) -> [Qmeas]
  [Pmeas] -> Mux1/2
  [Pref] -> Divide/1
  Demux/1 -> Divide/2
  Divide/1 -> Scope1/1, Saturation2/1
  [VdVq] -> Demux/1
  Saturation2/1 -> [Id_ref]
  Current Regulator (Ireg)/2(Uref_dq0) -> Goto9/1

== system P2PHVDCMMC/DC & converter 2 ==
  note: Cable (simplified model)
  CnDC : spsSeriesRLCBranchLib/Series RLC Branch  LConnTagsString=__new0  RConnTagsString=__new0  BranchType=RC  Resistance=Rg  Inductance=1e-3  SetiL0=off  InitialCurrent=0  Capacitance=Cg  Setx0=off  InitialVoltage=Vnom_dc/2  Measurements=None
  CpDC : spsSeriesRLCBranchLib/Series RLC Branch  LConnTagsString=__new0  RConnTagsString=__new0  BranchType=RC  Resistance=Rg  Inductance=1e-3  SetiL0=off  InitialCurrent=0  Capacitance=Cg  Setx0=off  InitialVoltage=Vnom_dc/2  Measurements=None
  Ground4 : spsGroundLib/Ground  LConnTagsString=a
  Subsystem : Subsystem
      settings: PortSchema="{\"entries\":[{\"content\":{\"sides\":[{\"content\":{},\"type\":\"ConnectorPlacement.EquallySpacedRectSide\",\"uuid\":\"4e02d665-d085-4b85-80a9-e764fc967845\"},{\"content\":{\"side\":\"RIGHT\"},\"type\":\"ConnectorPlacement.EquallySpacedRectSide\",\"uuid\":\"30de6932-84d3-45b2-9250-05848cfa24a7\"},{\"content\":{\"connectorIds\":[\"LConn1\"],\"side\":\"TOP\"},\"type\":\"ConnectorPlacement.EquallySpacedRectSide\",\"uuid\":\"b576265a-02ae-4a0d-b102-a95af34a8809\"},{\"content\":{\"connectorIds\":[\"RConn1\"],\"side\":\"BOTTOM\"},\"type\":\"ConnectorPlacement.EquallySpacedRectSide\",\"uuid\":\"0a0a1a6f-d60d-4cd9-8e89-b506a5f99912\"}]},\"type\":\"ConnectorPlacement.EquallySpacedConnector\",\"uuid\":\"a940d721-c0be-496a-91aa-f93d82b250c4\"}],\"packageUris\":[\"http://schema.mathworks.com/mf0/Connector/R2020b\"],\"version\":\"1.0\"}"
  Zcable1_1 : spsSeriesRLCBranchLib/Series RLC Branch  LConnTagsString=__new0  RConnTagsString=__new0  BranchType=RL  Resistance=R_cable/2  Inductance=L_cable/2  SetiL0=off  InitialCurrent=0  Capacitance=1e-6  Setx0=off  InitialVoltage=0  Measurements=None
  Zcable1_2 : spsSeriesRLCBranchLib/Series RLC Branch  LConnTagsString=__new0  RConnTagsString=__new0  BranchType=RL  Resistance=R_cable/2  Inductance=L_cable/2  SetiL0=off  InitialCurrent=0  Capacitance=1e-6  Setx0=off  InitialVoltage=0  Measurements=None
  Zcable2_1 : spsSeriesRLCBranchLib/Series RLC Branch  LConnTagsString=__new0  RConnTagsString=__new0  BranchType=RL  Resistance=R_cable/2  Inductance=L_cable/2  SetiL0=off  InitialCurrent=0  Capacitance=1e-6  Setx0=off  InitialVoltage=0  Measurements=None
  Zcable2_2 : spsSeriesRLCBranchLib/Series RLC Branch  LConnTagsString=__new0  RConnTagsString=__new0  BranchType=RL  Resistance=R_cable/2  Inductance=L_cable/2  SetiL0=off  InitialCurrent=0  Capacitance=1e-6  Setx0=off  InitialVoltage=0  Measurements=None
  1 : PMIOPort  Side=Left
  2 : PMIOPort  Port=2  Side=Left
  Connection Port : PMIOPort  Port=3  Side=Right
  Connection Port1 : PMIOPort  Port=4  Side=Right
  connections:
  Ground4/LConn1 -- CnDC/LConn1 -- CpDC/RConn1
  Subsystem/LConn1 -- Zcable1_1/RConn1 -- CpDC/LConn1 -- 1/RConn1
  CnDC/RConn1 -- 2/RConn1 -- Zcable2_1/RConn1 -- Subsystem/RConn1
  Zcable1_1/LConn1 -- Zcable1_2/RConn1
  Zcable2_2/RConn1 -- Zcable2_1/LConn1
  Connection Port/RConn1 -- Zcable1_2/LConn1
  Connection Port1/RConn1 -- Zcable2_2/LConn1

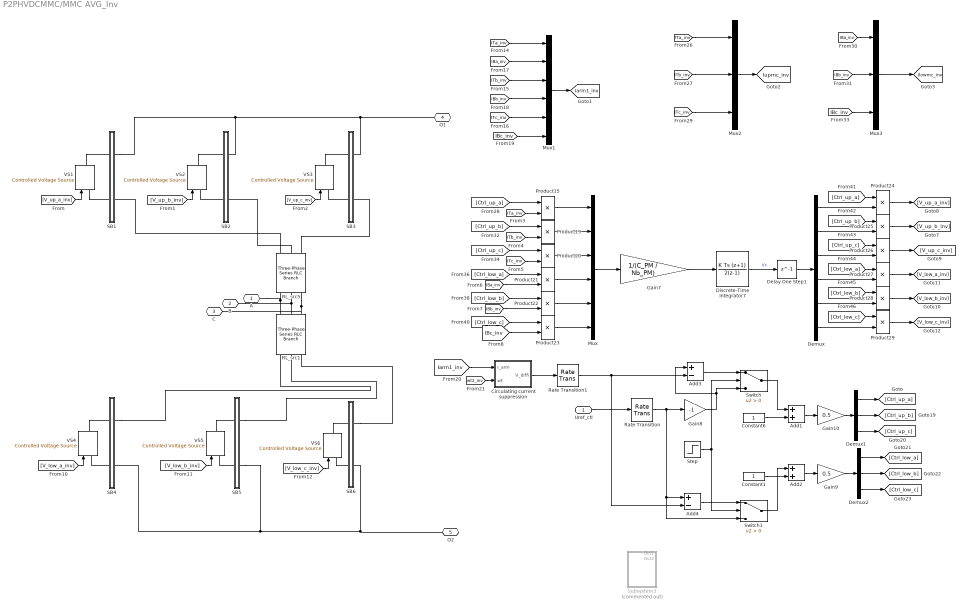
== system P2PHVDCMMC/MMC AVG_Inv ==
  Uref_ctl : Inport
  Add1 : Sum
  Add2 : Sum
  Add3 : Sum  Inputs=+-
  Add4 : Sum  Inputs=+-
  Circulating current suppression : Subsystem  VariantControl=Variant1
  Constant1 : Constant
  Constant6 : Constant
  Delay One Step1 : Delay  DelayLength=1
  Demux : Demux  Outputs=6
  Demux1 : Demux  Outputs=3
  Demux2 : Demux  Outputs=3
  Discrete-Time Integrator7 : DiscreteIntegrator  IntegratorMethod=Integration: Trapezoidal  gainval=1  SampleTime=Ts_Power  UpperSaturationLimit=5000  LowerSaturationLimit=500  ICPrevOutput=DiscIntNeverNeededParam  ICPrevScaledInput=DiscIntNeverNeededParam
  Gain10 : Gain  Gain=0.5
  Gain7 : Gain  Gain=1/(C_PM / Nb_PM)
  Gain8 : Gain  Gain=-1
  Gain9 : Gain  Gain=0.5
  Mux : Mux  Inputs=6
  Mux1 : Mux  Inputs=6
  Mux2 : Mux  Inputs=3
  Mux3 : Mux  Inputs=3
  Product{15,19..29} (12 alike) : Product
  RL_src1 : spsThreePhaseSeriesRLCBranchLib/Three-Phase Series RLC Branch  LConnTagsString=A|B|C  RConnTagsString=A|B|C  BranchType=RL  Resistance=Rarm  Inductance=Larm  Capacitance=1/(0.55*0.080*(500e3^2/100e6))/(2*pi*60)  Measurements=None
  RL_src5 : spsThreePhaseSeriesRLCBranchLib/Three-Phase Series RLC Branch  LConnTagsString=A|B|C  RConnTagsString=A|B|C  BranchType=RL  Resistance=Rarm  Inductance=Larm  Capacitance=1/(0.55*0.080*(500e3^2/100e6))/(2*pi*60)  Measurements=None
  Rate Transition : RateTransition  OutPortSampleTime=Ts_Power
  Rate Transition1 : RateTransition  OutPortSampleTime=Ts_Power
  SB1 : Subsystem
  SB2 : Subsystem
  SB3 : Subsystem
  SB4 : Subsystem
  SB5 : Subsystem
  SB6 : Subsystem
  Step : Step  Time=2  SampleTime=0
  Subsystem3 : Subsystem  Commented=on
  Switch : Switch  Criteria=u2 > Threshold  SaturateOnIntegerOverflow=off  InputSameDT=off
  Switch1 : Switch  Criteria=u2 > Threshold  SaturateOnIntegerOverflow=off  InputSameDT=off
  VS{1..6} (6 alike) : spsControlledVoltageSourceLib/Controlled Voltage Source  Initialize=on  Source_Type=AC  Amplitude=0  Phase=0  Frequency=0  Measurements=None
  A : PMIOPort  Side=Left
  B : PMIOPort  Port=2  Side=Left
  C : PMIOPort  Port=3  Side=Left
  O1 : PMIOPort  Port=4  Side=Right
  O2 : PMIOPort  Port=5  Side=Right
  tag scope: Iarm1_inv=global, Ilowmc_inv=global, Iupmc_inv=global
  wires:
  Add4/1 -> Switch1/1
  Gain8/1 -> Switch/3, Add3/1
  Add3/1 -> Switch/1
  Rate Transition1/1 -> Add4/2, Add3/2
  [IBa_inv] -> Mux1/2
  Circulating current suppression/1(V_diffi) -> Rate Transition1/1
  Mux1/1 -> [Iarm1_inv]
  [IBc_inv] -> Mux1/6
  [IBb_inv] -> Mux1/4
  Product29/1 -> [V_low_c_inv]
  Constant6/1 -> Add1/2
  Uref_ctl/1 -> Rate Transition/1
  Demux/5 -> Product28/2
  Demux2/2 -> [Ctrl_low_b]
  Product25/1 -> [V_up_b_inv]
  [Ctrl_low_b] -> Product22/1
  Product20/1 -> Mux/3
  Constant1/1 -> Add2/2
  [Ctrl_low_a] -> Product27/1
  Demux1/2 -> [Ctrl_up_b]
  [Ctrl_up_b] -> Product25/1
  Gain9/1 -> Demux2/1
  Demux/6 -> Product29/2
  Gain10/1 -> Demux1/1
  Demux/3 -> Product26/2
  [Ctrl_up_a] -> Product24/1
  Product28/1 -> [V_low_b_inv]
  Demux2/1 -> [Ctrl_low_a]
  [Ctrl_up_c] -> Product26/1
  Product23/1 -> Mux/6
  Demux1/3 -> [Ctrl_up_c]
  Product19/1 -> Mux/2
  [Ctrl_up_c] -> Product20/1
  [Ctrl_low_a] -> Product21/1
  [Ctrl_up_b] -> Product19/1
  [Ctrl_low_c] -> Product23/1
  [Ctrl_up_a] -> Product15/1
  Product27/1 -> [V_low_a_inv]
  Rate Transition/1 -> Gain8/1, Switch1/3, Add4/1
  Discrete-Time Integrator7/1 -> Delay One Step1/1  "Vc"
  Demux/4 -> Product27/2
  Add2/1 -> Gain9/1
  Product21/1 -> Mux/4
  Demux1/1 -> [Ctrl_up_a]
  Step/1 -> Switch/2, Switch1/2
  [ITa_inv] -> Mux1/1
  [ITc_inv] -> Mux1/5
  Product22/1 -> Mux/5
  Mux/1 -> Gain7/1
  Demux2/3 -> [Ctrl_low_c]
  Delay One Step1/1 -> Demux/1
  Product26/1 -> [V_up_c_inv]
  Demux/2 -> Product25/2
  [Ctrl_low_c] -> Product29/1
  Product15/1 -> Mux/1
  [Ctrl_low_b] -> Product28/1
  Product24/1 -> [V_up_a_inv]
  Add1/1 -> Gain10/1
  [wt2_inv] -> Circulating current suppression/2(wt)
  [ITb_inv] -> Mux1/3
  [Iarm1_inv] -> Circulating current suppression/1(I_arm)
  Demux/1 -> Product24/2
  Gain7/1 -> Discrete-Time Integrator7/1
  [V_up_c_inv] -> VS3/1
  [V_low_a_inv] -> VS4/1
  [V_up_a_inv] -> VS1/1
  [V_low_b_inv] -> VS5/1
  [V_up_b_inv] -> VS2/1
  [V_low_c_inv] -> VS6/1
  [ITa_inv] -> Product15/2
  [ITc_inv] -> Product20/2
  [ITb_inv] -> Product19/2
  [IBa_inv] -> Product21/2
  [IBb_inv] -> Product22/2
  [IBc_inv] -> Product23/2
  [ITb_inv] -> Mux2/2
  [ITc_inv] -> Mux2/3
  [ITa_inv] -> Mux2/1
  Mux2/1 -> [Iupmc_inv]
  [IBa_inv] -> Mux3/1
  [IBb_inv] -> Mux3/2
  [IBc_inv] -> Mux3/3
  Mux3/1 -> [Ilowmc_inv]
  Switch1/1 -> Add2/1
  Switch/1 -> Add1/1
  connections:
  VS1/LConn1 -- SB1/LConn2
  SB5/LConn2 -- VS5/LConn1
  RL_src5/LConn2 -- SB2/RConn2
  SB3/LConn1 -- VS3/RConn1
  SB4/LConn2 -- VS4/LConn1
  SB2/LConn1 -- VS2/RConn1
  SB5/RConn1 -- RL_src1/LConn2
  SB6/LConn1 -- VS6/RConn1
  SB6/RConn1 -- RL_src1/LConn3
  SB4/RConn1 -- RL_src1/LConn1
  VS1/RConn1 -- SB1/LConn1
  SB4/LConn1 -- VS4/RConn1
  RL_src5/LConn3 -- SB3/RConn2
  SB5/LConn1 -- VS5/RConn1
  VS6/LConn1 -- SB6/LConn2
  SB3/LConn2 -- VS3/LConn1
  SB2/LConn2 -- VS2/LConn1
  RL_src1/RConn1 -- A/RConn1 -- RL_src5/RConn1
  RL_src1/RConn2 -- RL_src5/RConn2 -- B/RConn1
  RL_src1/RConn3 -- RL_src5/RConn3 -- C/RConn1
  RL_src5/LConn1 -- SB1/RConn2
  SB3/RConn1 -- SB2/RConn1 -- SB1/RConn1 -- O1/RConn1
  O2/RConn1 -- SB6/RConn2 -- SB5/RConn2 -- SB4/RConn2

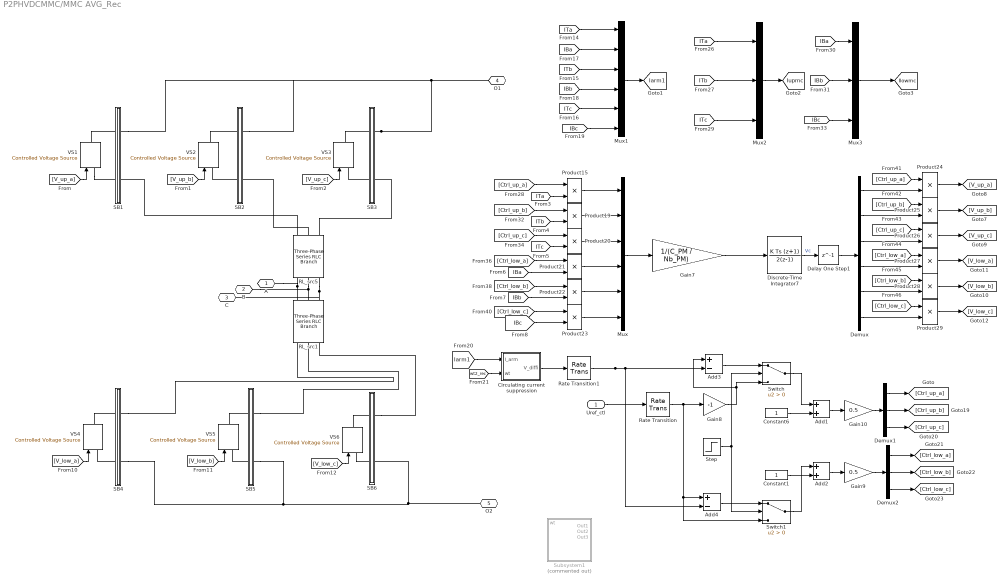
== system P2PHVDCMMC/MMC AVG_Rec ==
  Uref_ctl : Inport
  Add1 : Sum
  Add2 : Sum
  Add3 : Sum  Inputs=+-
  Add4 : Sum  Inputs=+-
  Circulating current suppression : Subsystem  VariantControl=Variant1
  Constant1 : Constant
  Constant6 : Constant
  Delay One Step1 : Delay  DelayLength=1
  Demux : Demux  Outputs=6
  Demux1 : Demux  Outputs=3
  Demux2 : Demux  Outputs=3
  Discrete-Time Integrator7 : DiscreteIntegrator  IntegratorMethod=Integration: Trapezoidal  gainval=1  SampleTime=Ts_Power  UpperSaturationLimit=5000  LowerSaturationLimit=500  ICPrevOutput=DiscIntNeverNeededParam  ICPrevScaledInput=DiscIntNeverNeededParam
  Gain10 : Gain  Gain=0.5
  Gain7 : Gain  Gain=1/(C_PM / Nb_PM)
  Gain8 : Gain  Gain=-1
  Gain9 : Gain  Gain=0.5
  Mux : Mux  Inputs=6
  Mux1 : Mux  Inputs=6
  Mux2 : Mux  Inputs=3
  Mux3 : Mux  Inputs=3
  Product{15,19..29} (12 alike) : Product
  RL_src1 : spsThreePhaseSeriesRLCBranchLib/Three-Phase Series RLC Branch  LConnTagsString=A|B|C  RConnTagsString=A|B|C  BranchType=RL  Resistance=Rarm  Inductance=Larm  Capacitance=1/(0.55*0.080*(500e3^2/100e6))/(2*pi*60)  Measurements=None
  RL_src5 : spsThreePhaseSeriesRLCBranchLib/Three-Phase Series RLC Branch  LConnTagsString=A|B|C  RConnTagsString=A|B|C  BranchType=RL  Resistance=Rarm  Inductance=Larm  Capacitance=1/(0.55*0.080*(500e3^2/100e6))/(2*pi*60)  Measurements=None
  Rate Transition : RateTransition  OutPortSampleTime=Ts_Power
  Rate Transition1 : RateTransition  OutPortSampleTime=Ts_Power
  SB1 : Subsystem
  SB2 : Subsystem
  SB3 : Subsystem
  SB4 : Subsystem
  SB5 : Subsystem
  SB6 : Subsystem
  Step : Step  Time=2  SampleTime=0
  Subsystem1 : Subsystem  Commented=on
  Switch : Switch  Criteria=u2 > Threshold  SaturateOnIntegerOverflow=off  InputSameDT=off
  Switch1 : Switch  Criteria=u2 > Threshold  SaturateOnIntegerOverflow=off  InputSameDT=off
  VS{1..6} (6 alike) : spsControlledVoltageSourceLib/Controlled Voltage Source  Initialize=on  Source_Type=AC  Amplitude=0  Phase=0  Frequency=0  Measurements=None
  A : PMIOPort  Side=Left
  B : PMIOPort  Port=2  Side=Left
  C : PMIOPort  Port=3  Side=Left
  O1 : PMIOPort  Port=4  Side=Right
  O2 : PMIOPort  Port=5  Side=Right
  tag scope: Iarm1=global, Ilowmc=global, Iupmc=global
  wires:
  Add4/1 -> Switch1/1
  Gain8/1 -> Switch/3, Add3/1
  Add3/1 -> Switch/1
  Rate Transition1/1 -> Add4/2, Add3/2
  [IBa] -> Mux1/2
  Circulating current suppression/1(V_diffi) -> Rate Transition1/1
  Mux1/1 -> [Iarm1]
  [IBc] -> Mux1/6
  [IBb] -> Mux1/4
  Product29/1 -> [V_low_c]
  Constant6/1 -> Add1/2
  Uref_ctl/1 -> Rate Transition/1
  Demux/5 -> Product28/2
  Demux2/2 -> [Ctrl_low_b]
  Product25/1 -> [V_up_b]
  [Ctrl_low_b] -> Product22/1
  Product20/1 -> Mux/3
  Constant1/1 -> Add2/2
  [Ctrl_low_a] -> Product27/1
  Demux1/2 -> [Ctrl_up_b]
  [Ctrl_up_b] -> Product25/1
  Gain9/1 -> Demux2/1
  Demux/6 -> Product29/2
  Gain10/1 -> Demux1/1
  Demux/3 -> Product26/2
  [Ctrl_up_a] -> Product24/1
  Product28/1 -> [V_low_b]
  Demux2/1 -> [Ctrl_low_a]
  [Ctrl_up_c] -> Product26/1
  Product23/1 -> Mux/6
  Demux1/3 -> [Ctrl_up_c]
  Product19/1 -> Mux/2
  [Ctrl_up_c] -> Product20/1
  [Ctrl_low_a] -> Product21/1
  [Ctrl_up_b] -> Product19/1
  [Ctrl_low_c] -> Product23/1
  [Ctrl_up_a] -> Product15/1
  Product27/1 -> [V_low_a]
  Rate Transition/1 -> Gain8/1, Switch1/3, Add4/1
  Discrete-Time Integrator7/1 -> Delay One Step1/1  "Vc"
  Demux/4 -> Product27/2
  Add2/1 -> Gain9/1
  Product21/1 -> Mux/4
  Demux1/1 -> [Ctrl_up_a]
  Step/1 -> Switch/2, Switch1/2
  [ITa] -> Mux1/1
  [ITc] -> Mux1/5
  Product22/1 -> Mux/5
  Mux/1 -> Gain7/1
  Demux2/3 -> [Ctrl_low_c]
  Delay One Step1/1 -> Demux/1
  Product26/1 -> [V_up_c]
  Demux/2 -> Product25/2
  [Ctrl_low_c] -> Product29/1
  Product15/1 -> Mux/1
  [Ctrl_low_b] -> Product28/1
  Product24/1 -> [V_up_a]
  Add1/1 -> Gain10/1
  [wt2_rec] -> Circulating current suppression/2(wt)
  [ITb] -> Mux1/3
  [Iarm1] -> Circulating current suppression/1(I_arm)
  Demux/1 -> Product24/2
  Gain7/1 -> Discrete-Time Integrator7/1
  [V_up_c] -> VS3/1
  [V_low_a] -> VS4/1
  [V_up_a] -> VS1/1
  [V_low_b] -> VS5/1
  [V_up_b] -> VS2/1
  [V_low_c] -> VS6/1
  [ITa] -> Product15/2
  [ITc] -> Product20/2
  [ITb] -> Product19/2
  [IBa] -> Product21/2
  [IBb] -> Product22/2
  [IBc] -> Product23/2
  [ITb] -> Mux2/2
  [ITc] -> Mux2/3
  [ITa] -> Mux2/1
  Mux2/1 -> [Iupmc]
  [IBa] -> Mux3/1
  [IBb] -> Mux3/2
  [IBc] -> Mux3/3
  Mux3/1 -> [Ilowmc]
  Switch1/1 -> Add2/1
  Switch/1 -> Add1/1
  connections:
  VS1/LConn1 -- SB1/LConn2
  SB5/LConn2 -- VS5/LConn1
  RL_src5/LConn2 -- SB2/RConn2
  SB3/LConn1 -- VS3/RConn1
  SB4/LConn2 -- VS4/LConn1
  SB2/LConn1 -- VS2/RConn1
  SB5/RConn1 -- RL_src1/LConn2
  SB6/LConn1 -- VS6/RConn1
  SB6/RConn1 -- RL_src1/LConn3
  SB4/RConn1 -- RL_src1/LConn1
  VS1/RConn1 -- SB1/LConn1
  SB4/LConn1 -- VS4/RConn1
  RL_src5/LConn3 -- SB3/RConn2
  SB5/LConn1 -- VS5/RConn1
  VS6/LConn1 -- SB6/LConn2
  SB3/LConn2 -- VS3/LConn1
  SB2/LConn2 -- VS2/LConn1
  RL_src1/RConn1 -- A/RConn1 -- RL_src5/RConn1
  RL_src1/RConn2 -- RL_src5/RConn2 -- B/RConn1
  RL_src1/RConn3 -- RL_src5/RConn3 -- C/RConn1
  RL_src5/LConn1 -- SB1/RConn2
  SB3/RConn1 -- O1/RConn1 -- SB2/RConn1 -- SB1/RConn1
  SB4/RConn2 -- SB5/RConn2 -- O2/RConn1 -- SB6/RConn2
